simulink model "PID_controller"  (R2020b)
settings: Solver=VariableStepAuto  StartTime=0.0  StopTime=10.0  RelTol=1e-3
model workspace (MAT data in the model file):
  Kd = 120
  Ki = 200
  Kp = 350
settings Model: Creator=varunraj  LastModifiedBy=varunraj
settings DataIOCC: SaveOutput=off  SaveTime=off

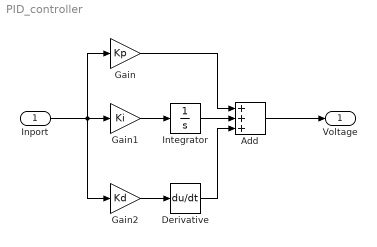
== system PID_controller ==
  Inport : Inport  OutDataTypeStr=double  PortDimensions=1  SampleTime=0
  Add : Sum  Inputs=+++
  Derivative : Derivative
  Gain : Gain  Gain=Kp
  Gain1 : Gain  Gain=Ki
  Gain2 : Gain  Gain=Kd
  Integrator : Integrator
  Voltage : Outport  OutDataTypeStr=double  PortDimensions=1  SampleTime=0
  wires:
  Integrator/1 -> Add/2
  Derivative/1 -> Add/3
  Add/1 -> Voltage/1
  Gain/1 -> Add/1
  Inport/1 -> Gain2/1, Gain/1, Gain1/1
  Gain2/1 -> Derivative/1
  Gain1/1 -> Integrator/1
